simulink model "drop_mech"  (Simulink 7.6)
settings: Solver=FixedStepDiscrete  StartTime=0.0  StopTime=0  RelTol=1e-3
settings Model: Creator=Administrator  LastModifiedBy=auvt
settings RTWCC: TargetLang=C++

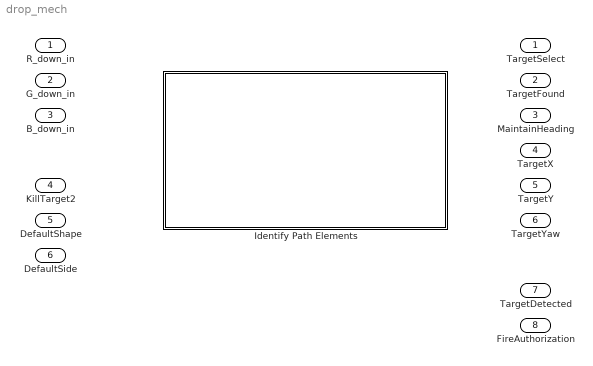
== system drop_mech ==
  R_down_in : Inport
  G_down_in : Inport  Port=2
  B_down_in : Inport  Port=3
  KillTarget2 : Inport  Port=4
  DefaultShape : Inport  Port=5
  DefaultSide : Inport  Port=6
  Identify Path Elements : Stateflow chart  TreatAsAtomicUnit=on  SystemSampleTime=[1/30 0]
  TargetSelect : Outport  OutDataTypeStr=double
  TargetFound : Outport  Port=2  OutDataTypeStr=double
  MaintainHeading : Outport  Port=3  OutDataTypeStr=double
  TargetX : Outport  Port=4  OutDataTypeStr=double
  TargetY : Outport  Port=5  OutDataTypeStr=double
  TargetYaw : Outport  Port=6  OutDataTypeStr=double
  TargetDetected : Outport  Port=7  OutDataTypeStr=double
  FireAuthorization : Outport  Port=8  OutDataTypeStr=double

== matlab function Identify Path Elements ==
function notes
%#eml

% Method 1
%  Scan all four bins left to right
%    could be as simple as progressive targeting; target one until over top
%      then target the next, etc.
%  Rely on well-balanced segmentation for black, white, and red
%  Classify each bin by:
%    shape
%      test center region for presence of true pixels
%      hough transform consider geometry of top 200 lines ("are there 4
%        lines that could constitute a box and an x?")
%      border energy analysis
%    blob (bbox xor area) determines relative size
%  Use strafing (or following) routines in model to get over top of correct
%    target
%  Throw fire authorization
%  Progress to second target
%  Throw fire authorization
%
%  Note: Realistically MUST be able to be entered at ANY point in the
%    process


return
